simulink model "Multi_Boiler_Common_header"  (R2025b)
settings: Solver=ode15s  StartTime=0.0  StopTime=800  FixedStep=1000  RelTol=1e-2
values from neighbouring files (symbols this model uses):
  Adc = 0.7    [Init_two_Boilers.m]
  b = 0.030    (= 0.03)    [Init_two_Boilers.m]
  k1 = (2 * rho_w1 * Adc * (rho_w1 - rho_s1) * g * a7_1 * Vr) / max(q_dc^2, 1e-12)    [Init_two_Boilers.m]
  k2 = (2 * rho_w2 * Adc * (rho_w2 - rho_s2) * g * a7_2 * Vr) / max(q_dc^2, 1e-12)    [Init_two_Boilers.m]
  m_metal = 1e6    (= 1000000)    [Init_two_Boilers.m]
  m_riser = 2e5    (= 200000)    [Init_two_Boilers.m]
  tau_s = 1e-2    (= 0.01)    [Init_two_Boilers.m]
  u0_1 = [Q1_MW; q_s1; q_s1; h_f]    [Init_two_Boilers.m]
  u0_2 = [Q2_MW; q_s2; q_s2; h_f]    [Init_two_Boilers.m]
  Vr = 37    [Init_two_Boilers.m]
libraries: slpidlib x4
settings Model: SimulationMode=accelerator  PacingRate=9  Creator=Zwivh  LastModifiedBy=Zwivh
settings DebuggingCC: AlgebraicLoopMsg=none

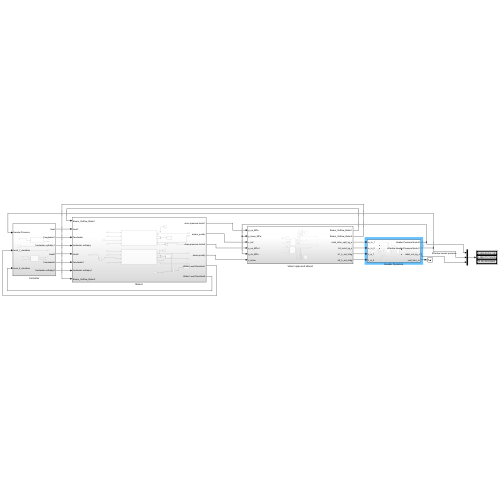
[thumbnail: Simulink's stored preview of the top-level diagram]
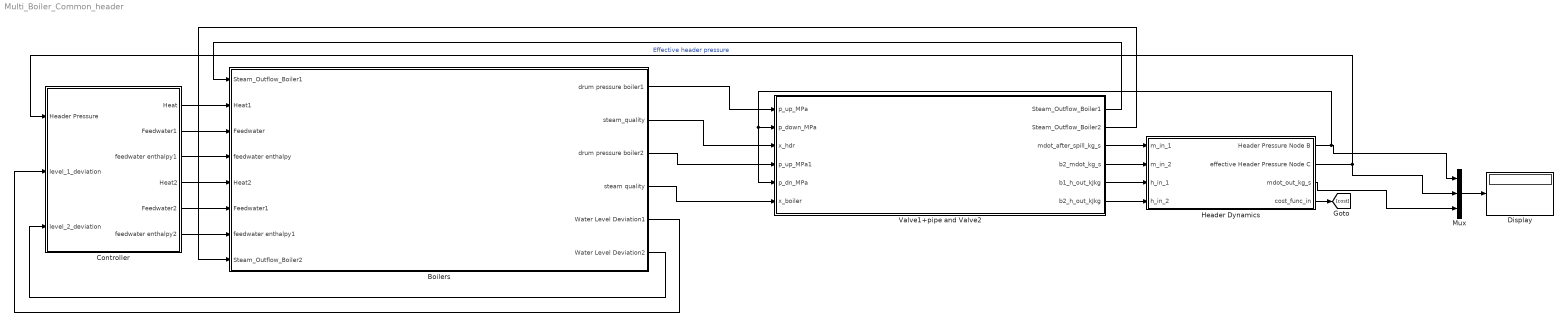
== system Multi_Boiler_Common_header ==
  Boilers : Subsystem
  Controller : Subsystem
  Display : Display
  Header Dynamics : Subsystem
  Mux : Mux  Inputs=3
  Valve1+pipe and Valve2 : Subsystem
  wires:
  Boilers/1(drum pressure boiler1) -> Valve1+pipe and Valve2/1(p_up_MPa)
  Boilers/2(steam_quality) -> Valve1+pipe and Valve2/3(x_hdr)
  Boilers/3(drum pressure boiler2) -> Valve1+pipe and Valve2/4(p_up_MPa1)
  Boilers/4(steam quality) -> Valve1+pipe and Valve2/6(x_boiler)
  Valve1+pipe and Valve2/1(Steam_Outflow_Boiler1) -> Boilers/1(Steam_Outflow_Boiler1)
  Valve1+pipe and Valve2/2(Steam_Outflow_Boiler2) -> Boilers/8(Steam_Outflow_Boiler2)
  Controller/1(Heat) -> Boilers/2(Heat1)
  Controller/2(Feedwater1) -> Boilers/3(Feedwater)
  Controller/3(feedwater enthalpy1) -> Boilers/4(feedwater enthalpy)
  Controller/4(Heat2) -> Boilers/5(Heat2)
  Controller/5(Feedwater2) -> Boilers/6(Feedwater1)
  Controller/6(feedwater enthalpy2) -> Boilers/7(feedwater enthalpy1)
  Valve1+pipe and Valve2/4(b2_mdot_kg_s) -> Header Dynamics/2(m_in_2)
  Valve1+pipe and Valve2/5(b1_h_out_kJkg) -> Header Dynamics/3(h_in_1)
  Valve1+pipe and Valve2/6(b2_h_out_kJkg) -> Header Dynamics/4(h_in_2)
  Mux/1 -> Display/1
  Header Dynamics/1(Header Pressure Node B) -> Mux/1, Valve1+pipe and Valve2/5(p_dn_MPa), Valve1+pipe and Valve2/2(p_down_MPa)
  Header Dynamics/3(mdot_out_kg_s) -> Mux/3
  Header Dynamics/2(effective Header Pressure Node C) -> Mux/2, Controller/1(Header Pressure)  "Effective header pressure"
  Header Dynamics/4(cost_func_in) -> [cost]
  Boilers/6(Water Level Deviation2) -> Controller/3(level_2_deviation)
  Boilers/5(Water Level Deviation1) -> Controller/2(level_1_deviation)
  Valve1+pipe and Valve2/3(mdot_after_spill_kg_s) -> Header Dynamics/1(m_in_1)

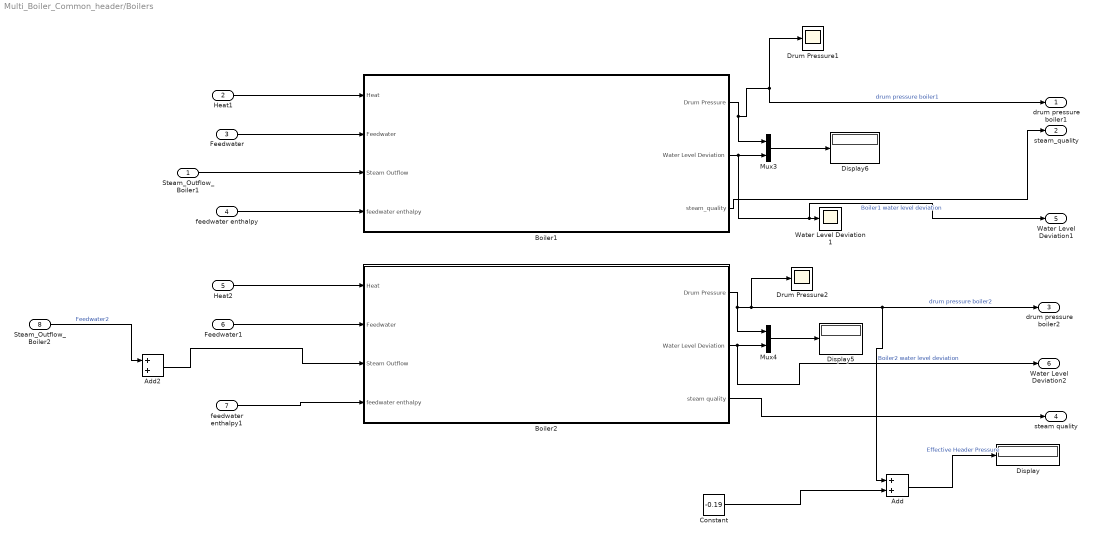
== system Multi_Boiler_Common_header/Boilers ==
  Steam_Outflow_Boiler1 : Inport
  Heat1 : Inport  Port=2
  Feedwater : Inport  Port=3
  feedwater enthalpy : Inport  Port=4
  Heat2 : Inport  Port=5
  Feedwater1 : Inport  Port=6
  feedwater enthalpy1 : Inport  Port=7
  Steam_Outflow_Boiler2 : Inport  Port=8
  Add : Sum
  Add2 : Sum
  Boiler1 : Subsystem
  Boiler2 : Subsystem
  Constant : Constant  Value=-0.19
  Display : Display
  Display5 : Display
  Display6 : Display
  Drum Pressure1 : Scope
      settings: ActiveDisplayYMinimum=2.409582484950084  ActiveDisplayYMaximum=65.31375763544925  DataLoggingVariableName=ScopeData7
  Drum Pressure2 : Scope
      settings: DataLoggingVariableName=ScopeData11
  Mux3 : Mux  Inputs=2
  Mux4 : Mux  Inputs=2
  Water Level Deviation 1 : Scope
      settings: DataLoggingVariableName=ScopeData10
  drum pressure boiler1 : Outport
  steam_quality : Outport  Port=2
  drum pressure boiler2 : Outport  Port=3
  steam quality : Outport  Port=4
  Water Level Deviation1 : Outport  Port=5
  Water Level Deviation2 : Outport  Port=6
  wires:
  Feedwater/1 -> Boiler1/2(Feedwater)
  Boiler1/1(Drum Pressure) -> Mux3/1, drum pressure boiler1/1, Drum Pressure1/1  "drum pressure boiler1"
  Boiler1/2(Water Level Deviation) -> Water Level Deviation1/1, Water Level Deviation 1/1, Mux3/2  "Boiler1 water level deviation"
  Steam_Outflow_Boiler1/1 -> Boiler1/3(Steam Outflow)
  Boiler2/2(Water Level Deviation) -> Water Level Deviation2/1, Mux4/2  "Boiler2 water level deviation"
  Mux3/1 -> Display6/1
  Feedwater1/1 -> Boiler2/2(Feedwater)
  feedwater enthalpy/1 -> Boiler1/4(feedwater enthalpy)
  Mux4/1 -> Display5/1
  Boiler2/3(steam quality) -> steam quality/1
  Boiler2/1(Drum Pressure) -> Mux4/1, Add/1, drum pressure boiler2/1, Drum Pressure2/1  "drum pressure boiler2"
  feedwater enthalpy1/1 -> Boiler2/4(feedwater enthalpy)
  Heat2/1 -> Boiler2/1(Heat)
  Heat1/1 -> Boiler1/1(Heat)
  Boiler1/3(steam_quality) -> steam_quality/1
  Add2/1 -> Boiler2/3(Steam Outflow)
  Steam_Outflow_Boiler2/1 -> Add2/1  "Feedwater2"
  Constant/1 -> Add/2
  Add/1 -> Display/1  "Effective Header Pressure"

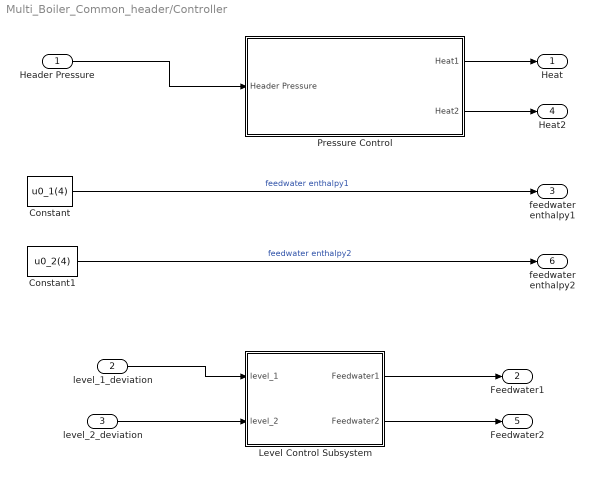
== system Multi_Boiler_Common_header/Controller ==
  Header Pressure : Inport
  level_1_deviation : Inport  Port=2
  level_2_deviation : Inport  Port=3
  Constant : Constant  Value=u0_1(4)
  Constant1 : Constant  Value=u0_2(4)
  Level Control Subsystem : Subsystem
  Pressure Control : Subsystem
  Heat : Outport
  Feedwater1 : Outport  Port=2
  feedwater enthalpy1 : Outport  Port=3
  Heat2 : Outport  Port=4
  Feedwater2 : Outport  Port=5
  feedwater enthalpy2 : Outport  Port=6
  wires:
  Constant1/1 -> feedwater enthalpy2/1  "feedwater enthalpy2"
  Constant/1 -> feedwater enthalpy1/1  "feedwater enthalpy1"
  Pressure Control/1(Heat1) -> Heat/1
  Pressure Control/2(Heat2) -> Heat2/1
  Level Control Subsystem/1(Feedwater1) -> Feedwater1/1
  Level Control Subsystem/2(Feedwater2) -> Feedwater2/1
  Header Pressure/1 -> Pressure Control/1(Header Pressure)
  level_2_deviation/1 -> Level Control Subsystem/2(level_2)
  level_1_deviation/1 -> Level Control Subsystem/1(level_1)

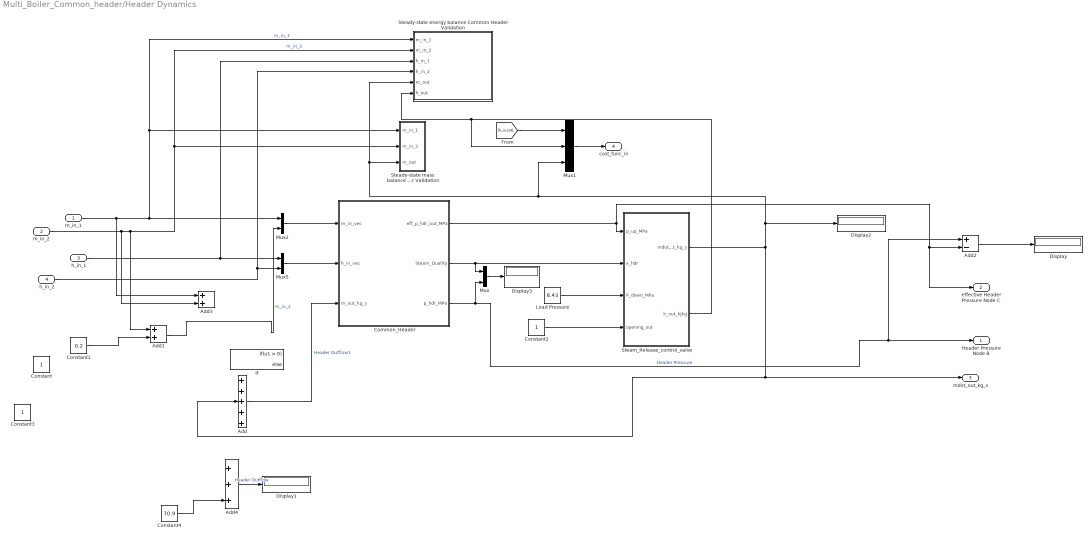
== system Multi_Boiler_Common_header/Header Dynamics ==
  m_in_1 : Inport
  m_in_2 : Inport  Port=2
  h_in_1 : Inport  Port=3
  h_in_2 : Inport  Port=4
  Add : Sum  Inputs=+++++
  Add1 : Sum
  Add2 : Sum  Inputs=+-
  Add3 : Sum
  Add4 : Sum  Inputs=+++
  Common_Header : Subsystem
  Constant : Constant
  Constant1 : Constant  Value=0.2
  Constant2 : Constant
  Constant3 : Constant
  Constant4 : Constant  Value=70.9
  Display{,1..3} (4 alike) : Display
  If : If
  Load Pressure : Constant  Value=8.43
  Mux : Mux  Inputs=2
  Mux1 : Mux  Inputs=3
  Mux2 : Mux  Inputs=2
  Mux5 : Mux  Inputs=2
  Steady‑state energy balance Common Header Validation : Subsystem
  Steady‑state mass balance Common Header Validation : Subsystem
  "Steam_Release_control_valve " : Subsystem
  Header Pressure Node B : Outport
  effective Header Pressure Node C : Outport  Port=2
  mdot_out_kg_s : Outport  Port=3
  cost_func_in : Outport  Port=4
  wires:
  Mux2/1 -> Common_Header/1(m_in_vec)
  Common_Header/2(Steam_Quality) -> Mux/1, "Steam_Release_control_valve "/2(x_hdr)
  "Steam_Release_control_valve "/2(h_out_kJkg) -> Mux1/2, Steady‑state energy balance Common Header Validation/6(h_out)
  m_in_1/1 -> Add3/1, Mux2/1, Steady‑state energy balance Common Header Validation/1(m_in_1), Steady‑state mass balance Common Header Validation/1(m_in_1)  "m_in_1"
  Mux5/1 -> Common_Header/2(h_in_vec)
  Load Pressure/1 -> "Steam_Release_control_valve "/3(P_down_MPa)
  Add/1 -> Common_Header/3(m_out_kg_s)  "Header Outflow1"
  Constant2/1 -> "Steam_Release_control_valve "/4(opening_out)
  h_in_1/1 -> Mux5/1, Steady‑state energy balance Common Header Validation/3(h_in_1)
  h_in_2/1 -> Mux5/2, Steady‑state energy balance Common Header Validation/4(h_in_2)
  m_in_2/1 -> Add3/2, Add1/1, Steady‑state energy balance Common Header Validation/2(m_in_2), Steady‑state mass balance Common Header Validation/2(m_in_2)  "m_in_2"
  Common_Header/1(eff_p_hdr_out_MPa) -> "Steam_Release_control_valve "/1(p_up_MPa), Add2/2, effective Header Pressure Node C/1
  Common_Header/3(p_hdr_MPa) -> Mux/2, Add2/1, Header Pressure Node B/1  "Header Pressure"
  Add2/1 -> Display/1
  Mux/1 -> Display3/1
  Mux1/1 -> cost_func_in/1
  [h_in_tot] -> Mux1/1
  Constant1/1 -> Add1/2
  Add1/1 -> Mux2/2  "m_in_2"
  "Steam_Release_control_valve "/1(mdot_out_kg_s) -> mdot_out_kg_s/1, Add/3, Mux1/3, Steady‑state energy balance Common Header Validation/5(m_out), Steady‑state mass balance Common Header Validation/3(m_out), Display2/1
  Constant4/1 -> Add4/3
  Add4/1 -> Display1/1  "Header Outflow"

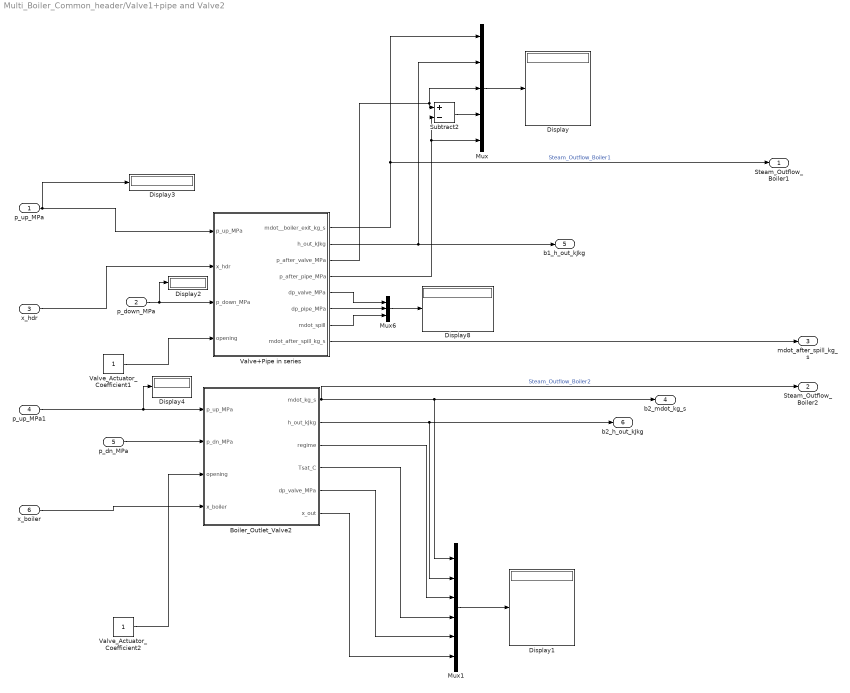
== system Multi_Boiler_Common_header/Valve1+pipe and Valve2 ==
  p_up_MPa : Inport
  p_down_MPa : Inport  Port=2
  x_hdr : Inport  Port=3
  p_up_MPa1 : Inport  Port=4
  p_dn_MPa : Inport  Port=5
  x_boiler : Inport  Port=6
  Boiler_Outlet_Valve2 : Subsystem
  Display{,1..4,8} (6 alike) : Display
  Mux : Mux  Inputs=5
  Mux1 : Mux  Inputs=6
  Mux6 : Mux  Inputs=3
  Subtract2 : Sum  Inputs=+-
  Valve+Pipe in series : Subsystem
  Valve_Actuator_Coefficient1 : Constant
  Valve_Actuator_Coefficient2 : Constant
  Steam_Outflow_Boiler1 : Outport
  Steam_Outflow_Boiler2 : Outport  Port=2
  mdot_after_spill_kg_s : Outport  Port=3
  b2_mdot_kg_s : Outport  Port=4
  b1_h_out_kJkg : Outport  Port=5
  b2_h_out_kJkg : Outport  Port=6
  wires:
  x_hdr/1 -> Valve+Pipe in series/2(x_hdr)
  Boiler_Outlet_Valve2/4(Tsat_C) -> Mux1/4
  Valve+Pipe in series/1(mdot__boiler_exit_kg_s) -> Mux/1, Steam_Outflow_Boiler1/1  "Steam_Outflow_Boiler1"
  Valve+Pipe in series/5(dp_valve_MPa) -> Mux6/1
  x_boiler/1 -> Boiler_Outlet_Valve2/4(x_boiler)
  Valve+Pipe in series/3(p_after_valve_MPa) -> Mux/3, Subtract2/1
  Valve+Pipe in series/4(p_after_pipe_MPa) -> Subtract2/2, Mux/5
  Valve_Actuator_Coefficient2/1 -> Boiler_Outlet_Valve2/3(opening)
  Mux1/1 -> Display1/1
  Boiler_Outlet_Valve2/2(h_out_kJkg) -> b2_h_out_kJkg/1, Mux1/2
  Mux/1 -> Display/1
  Boiler_Outlet_Valve2/6(x_out) -> Mux1/6
  Valve_Actuator_Coefficient1/1 -> Valve+Pipe in series/4(opening)
  Boiler_Outlet_Valve2/3(regime) -> Mux1/3
  Boiler_Outlet_Valve2/1(mdot_kg_s) -> b2_mdot_kg_s/1, Mux1/1, Steam_Outflow_Boiler2/1  "Steam_Outflow_Boiler2"
  Mux6/1 -> Display8/1
  Boiler_Outlet_Valve2/5(dp_valve_MPa) -> Mux1/5
  Subtract2/1 -> Mux/4
  Valve+Pipe in series/6(dp_pipe_MPa) -> Mux6/2
  Valve+Pipe in series/7(mdot_spill) -> Mux6/3
  Valve+Pipe in series/2(h_out_kJkg) -> b1_h_out_kJkg/1, Mux/2
  p_dn_MPa/1 -> Boiler_Outlet_Valve2/2(p_dn_MPa)
  p_down_MPa/1 -> Display2/1, Valve+Pipe in series/3(p_down_MPa)
  p_up_MPa/1 -> Display3/1, Valve+Pipe in series/1(p_up_MPa)
  p_up_MPa1/1 -> Display4/1, Boiler_Outlet_Valve2/1(p_up_MPa)
  Valve+Pipe in series/8(mdot_after_spill_kg_s) -> mdot_after_spill_kg_s/1

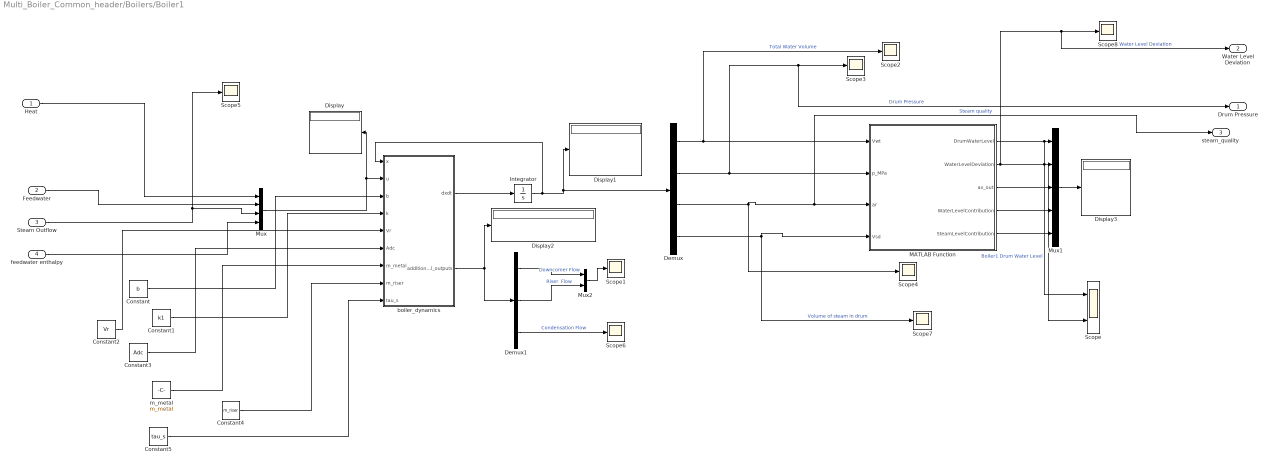
== system Multi_Boiler_Common_header/Boilers/Boiler1 ==
  Heat : Inport
  Feedwater : Inport  Port=2
  Steam Outflow : Inport  Port=3
  feedwater enthalpy : Inport  Port=4
  Constant : Constant  Value=b
  Constant1 : Constant  Value=k1
  Constant2 : Constant  Value=Vr
  Constant3 : Constant  Value=Adc
  Constant4 : Constant  Value=m_riser
  Constant5 : Constant  Value=tau_s
  Demux : Demux
  Demux1 : Demux  Outputs=3
  Display{,1..3} (4 alike) : Display
  Integrator : Integrator  InitialCondition=[57.8;8.8;0.083;4.9]
  MATLAB Function : MATLAB Function  TreatAsAtomicUnit=on
  Mux : Mux
  Mux1 : Mux  Inputs=5
  Mux2 : Mux  Inputs=2
  Scope : Scope  NumInputPorts=2
      settings: ActiveDisplayYMinimum=-0.11553187271684388  ActiveDisplayYMaximum=0.97989716685186512  DataLoggingVariableName=ScopeData9
  Scope{1..8} (8 alike) : Scope
      Scope1 settings: ActiveDisplayYMinimum=1149.8937170235527  ActiveDisplayYMaximum=1360.0825647224879  DataLoggingVariableName=ScopeData6
      Scope3 settings: ActiveDisplayYMinimum=5.1731172032500083  ActiveDisplayYMaximum=8.869653644083332
      Scope4 settings: DataLoggingVariableName=ScopeData2
      Scope5 settings: ActiveDisplayYMinimum=81.783639946245515  ActiveDisplayYMaximum=87.68969538020076  DataLoggingVariableName=ScopeData3
      Scope6 settings: DataLoggingVariableName=ScopeData4
      Scope7 settings: DataLoggingVariableName=ScopeData5
      Scope8 settings: ActiveDisplayYMinimum=-0.31931831052985321  ActiveDisplayYMaximum=0.12332586369569878  DataLoggingVariableName=ScopeData8
  boiler_dynamics : MATLAB Function  TreatAsAtomicUnit=on
  "m_metal " : Constant  Value=m_metal
  Drum Pressure : Outport
  Water Level Deviation : Outport  Port=2
  steam_quality : Outport  Port=3
  wires:
  MATLAB Function/3(av_out) -> Mux1/3
  Steam Outflow/1 -> Scope5/1, Mux/3
  Integrator/1 -> Display1/1, Demux/1, boiler_dynamics/1(x)
  Constant4/1 -> boiler_dynamics/8(m_riser)
  Demux/1 -> Scope2/1, MATLAB Function/1(Vwt)  "Total Water Volume"
  MATLAB Function/2(WaterLevelDeviation) -> Water Level Deviation/1, Scope8/1, Scope/2, Mux1/2  "Water Level Deviation"
  Demux/2 -> Drum Pressure/1, Scope3/1, MATLAB Function/2(p_MPa)  "Drum Pressure"
  Demux1/2 -> Mux2/2  "Riser  Flow"
  boiler_dynamics/2(additional_outputs) -> Display2/1, Demux1/1
  Constant2/1 -> boiler_dynamics/5(Vr)
  Demux/3 -> Scope4/1, steam_quality/1, MATLAB Function/3(ar)  "Steam quality"
  Constant3/1 -> boiler_dynamics/6(Adc)
  Mux2/1 -> Scope1/1
  Demux1/1 -> Mux2/1  "Downcomer Flow"
  Constant1/1 -> boiler_dynamics/4(k)
  Mux/1 -> Display/1, boiler_dynamics/2(u)
  MATLAB Function/5(SteamLevelContribution) -> Mux1/5
  MATLAB Function/1(DrumWaterLevel) -> Scope/1, Mux1/1  "Boiler1 Drum Water Level"
  Constant/1 -> boiler_dynamics/3(b)
  "m_metal "/1 -> boiler_dynamics/7(m_metal)
  Demux/4 -> Scope7/1, MATLAB Function/4(Vsd)  "Volume of steam in drum"
  Constant5/1 -> boiler_dynamics/9(tau_s)
  Heat/1 -> Mux/1
  boiler_dynamics/1(dxdt) -> Integrator/1
  Demux1/3 -> Scope6/1  "Condensation Flow"
  MATLAB Function/4(WaterLevelContribution) -> Mux1/4
  Mux1/1 -> Display3/1
  Feedwater/1 -> Mux/2
  feedwater enthalpy/1 -> Mux/4

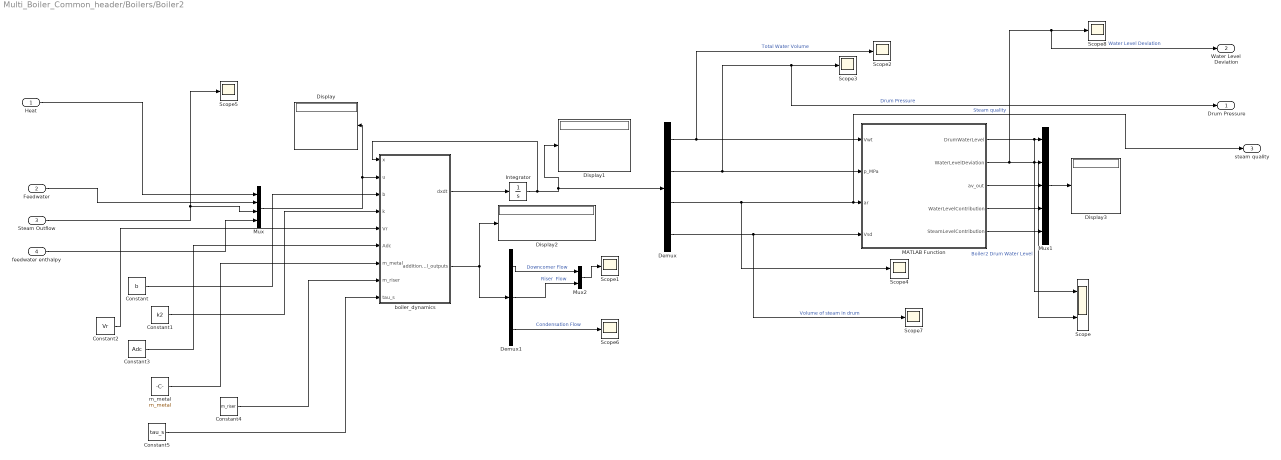
== system Multi_Boiler_Common_header/Boilers/Boiler2 ==
  Heat : Inport
  Feedwater : Inport  Port=2
  Steam Outflow : Inport  Port=3
  feedwater enthalpy : Inport  Port=4
  Constant : Constant  Value=b
  Constant1 : Constant  Value=k2
  Constant2 : Constant  Value=Vr
  Constant3 : Constant  Value=Adc
  Constant4 : Constant  Value=m_riser
  Constant5 : Constant  Value=tau_s
  Demux : Demux
  Demux1 : Demux  Outputs=3
  Display{,1..3} (4 alike) : Display
  Integrator : Integrator  InitialCondition=[57.6;8.69;0.066;4.9]
  MATLAB Function : MATLAB Function  TreatAsAtomicUnit=on
  Mux : Mux
  Mux1 : Mux  Inputs=5
  Mux2 : Mux  Inputs=2
  Scope : Scope  NumInputPorts=2
      settings: ActiveDisplayYMinimum=-0.43318786127461034  ActiveDisplayYMaximum=1.0681425276889893  DataLoggingVariableName=ScopeData9
  Scope{1..8} (8 alike) : Scope
      Scope1 settings: ActiveDisplayYMinimum=1149.8937170235527  ActiveDisplayYMaximum=1360.0825647224879  DataLoggingVariableName=ScopeData6
      Scope3 settings: ActiveDisplayYMinimum=7.2515160346094891  ActiveDisplayYMaximum=9.62463808005422
      Scope4 settings: DataLoggingVariableName=ScopeData2
      Scope5 settings: ActiveDisplayYMinimum=81.783639946245515  ActiveDisplayYMaximum=87.68969538020076  DataLoggingVariableName=ScopeData3
      Scope6 settings: DataLoggingVariableName=ScopeData4
      Scope7 settings: DataLoggingVariableName=ScopeData5
      Scope8 settings: ActiveDisplayYMinimum=-0.1700298535717597  ActiveDisplayYMaximum=0.091752188934218326  DataLoggingVariableName=ScopeData8
  boiler_dynamics : MATLAB Function  TreatAsAtomicUnit=on
  "m_metal " : Constant  Value=m_metal
  Drum Pressure : Outport
  Water Level Deviation : Outport  Port=2
  steam quality : Outport  Port=3
  wires:
  MATLAB Function/3(av_out) -> Mux1/3
  Steam Outflow/1 -> Scope5/1, Mux/3
  Integrator/1 -> Display1/1, Demux/1, boiler_dynamics/1(x)
  Constant4/1 -> boiler_dynamics/8(m_riser)
  Demux/1 -> Scope2/1, MATLAB Function/1(Vwt)  "Total Water Volume"
  MATLAB Function/2(WaterLevelDeviation) -> Water Level Deviation/1, Scope8/1, Scope/2, Mux1/2  "Water Level Deviation"
  Demux/2 -> Drum Pressure/1, Scope3/1, MATLAB Function/2(p_MPa)  "Drum Pressure"
  Demux1/2 -> Mux2/2  "Riser  Flow"
  boiler_dynamics/2(additional_outputs) -> Display2/1, Demux1/1
  Constant2/1 -> boiler_dynamics/5(Vr)
  Demux/3 -> Scope4/1, steam quality/1, MATLAB Function/3(ar)  "Steam quality"
  Constant3/1 -> boiler_dynamics/6(Adc)
  Mux2/1 -> Scope1/1
  Demux1/1 -> Mux2/1  "Downcomer Flow"
  Constant1/1 -> boiler_dynamics/4(k)
  Mux/1 -> Display/1, boiler_dynamics/2(u)
  MATLAB Function/5(SteamLevelContribution) -> Mux1/5
  MATLAB Function/1(DrumWaterLevel) -> Scope/1, Mux1/1  "Boiler2 Drum Water Level"
  Constant/1 -> boiler_dynamics/3(b)
  "m_metal "/1 -> boiler_dynamics/7(m_metal)
  Demux/4 -> Scope7/1, MATLAB Function/4(Vsd)  "Volume of steam in drum"
  Constant5/1 -> boiler_dynamics/9(tau_s)
  Heat/1 -> Mux/1
  boiler_dynamics/1(dxdt) -> Integrator/1
  Demux1/3 -> Scope6/1  "Condensation Flow"
  MATLAB Function/4(WaterLevelContribution) -> Mux1/4
  Mux1/1 -> Display3/1
  Feedwater/1 -> Mux/2
  feedwater enthalpy/1 -> Mux/4

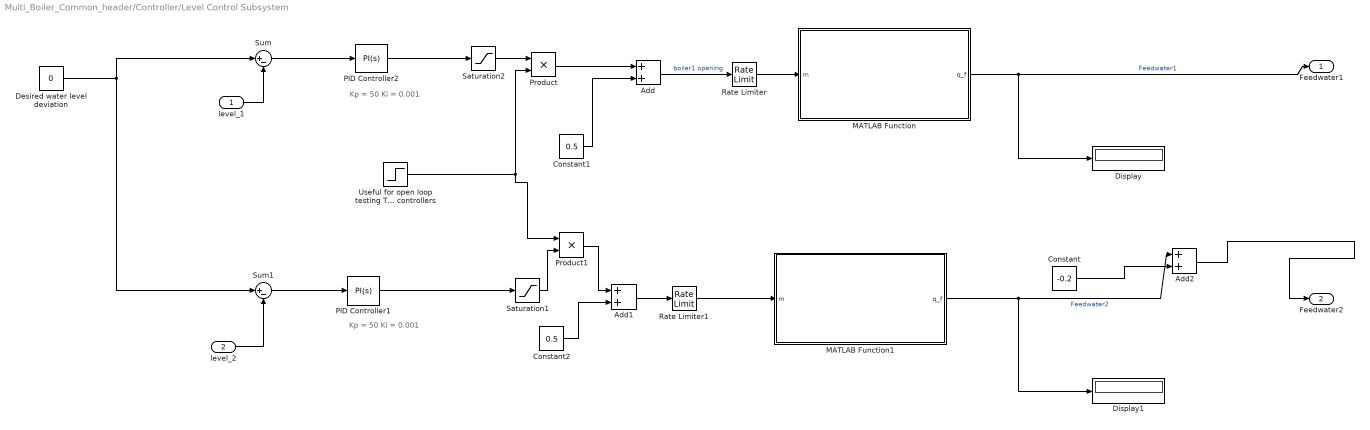
== system Multi_Boiler_Common_header/Controller/Level Control Subsystem ==
  note: Kp = 50
      | Ki = 0.001
  note: Kp = 50
      | Ki = 0.001
  level_1 : Inport
  level_2 : Inport  Port=2
  Add : Sum
  Add1 : Sum
  Add2 : Sum
  Constant : Constant  Value=-0.2
  Constant1 : Constant  Value=0.5
  Constant2 : Constant  Value=0.5
  "Desired water level deviation " : Constant  Value=0
  Display : Display
  Display1 : Display
  MATLAB Function : MATLAB Function  TreatAsAtomicUnit=on
  MATLAB Function1 : MATLAB Function  TreatAsAtomicUnit=on
  PID Controller1 : slpidlib/PID Controller  Controller=PI  Form=Parallel  TimeDomain=Continuous-time  UseExternalTs=off  SampleTime=5  IntegratorMethod=Forward Euler  FilterMethod=Forward Euler  ControllerParametersSource=internal  P=0.5e2  I=1e-3  UseKiTs=off  D=1  UseExternalDerivativeSource=off  N=100  UseFilter=on  TunerSelectOption=Transfer Function Based (PID Tuner App)  InitialConditionSource=internal  InitialConditionForIntegrator=0  InitialConditionForFilter=0  DifferentiatorICPrevScaledInput=0  ExternalReset=none  TrackingMode=off  Kt=1  LimitOutput=off  SatLimitsSource=internal  UpperSaturationLimit=inf  LowerSaturationLimit=-inf  LinearizeAsGain=on  AntiWindupMode=none  Kb=1  LimitIntegrator=off  UpperIntegratorSaturationLimit=inf  LowerIntegratorSaturationLimit=-inf  POutMin=[]  POutMax=[]  IOutMin=[]  IOutMax=[]  DOutMin=[]  DOutMax=[]  NOutMin=[]  NOutMax=[]  SumOutMin=[]  SumOutMax=[]  SaturationOutMin=[]  SaturationOutMax=[]  PParamMin=[]  PParamMax=[]  IParamMin=[]  IParamMax=[]  DParamMin=[]  DParamMax=[]  NParamMin=[]  NParamMax=[]  KbParamMin=[]  KbParamMax=[]  KtParamMin=[]  KtParamMax=[]  KbOutMin=[]  KbOutMax=[]  KtOutMin=[]  KtOutMax=[]  IntegratorOutMin=[]  IntegratorOutMax=[]  FilterOutMin=[]  FilterOutMax=[]  SumI1OutMin=[]  SumI1OutMax=[]  SumI2OutMin=[]  SumI2OutMax=[]  SumI3OutMin=[]  SumI3OutMax=[]  SumI4OutMin=[]  SumI4OutMax=[]  SumDOutMin=[]  SumDOutMax=[]  DifferentiatorOutMin=[]  DifferentiatorOutMax=[]  FilterDiffOutCoefMin=[]  FilterDiffOutCoefMax=[]  ReciprocalOutMin=[]  ReciprocalOutMax=[]  SumDenOutMin=[]  SumDenOutMax=[]  SumNumOutMin=[]  SumNumOutMax=[]  DivideOutMin=[]  DivideOutMax=[]  UdiffTsProdOutMin=[]  UdiffTsProdOutMax=[]  NTsProdOutMin=[]  NTsProdOutMax=[]  UintegralTsProdOutMin=[]  UintegralTsProdOutMax=[]  UngainTsProdOutMin=[]  UngainTsProdOutMax=[]  ClampingZeroOutDataTypeStr=Inherit: Inherit via back propagation  ClampingZeroOutMin=[]  ClampingZeroOutMax=[]  FilterDenConstantOutDataTypeStr=Inherit: Inherit via back propagation  FilterDenConstantOutMin=[]  FilterDenConstantOutMax=[]  PCopyOutDataTypeStr=Inherit: Inherit via back propagation  PCopyOutMin=[]  PCopyOutMax=[]  NCopyOutDataTypeStr=Inherit: Inherit via back propagation  NCopyOutMin=[]  NCopyOutMax=[]  IntegratorContinuousStateAttributes=''  IntegratorStateMustResolveToSignalObject=off  IntegratorRTWStateStorageClass=Auto  FilterContinuousStateAttributes=''  FilterStateMustResolveToSignalObject=off  FilterRTWStateStorageClass=Auto  ParallelPVariant=InternalParameters  IdealPVariant=Disabled  IVariant=InternalParameters  DVariant=Disabled  IntegratorVariant=Continuous  SatVariant=Disabled  AWVariant=Passthrough  PCopyVariant=Disabled  TRVariant=Disabled  FdbkBlocksVariant=Forward  IdealPFdbkVariant=Disabled  SatFdbkVariant=Disabled  DerivativeFilterVariant=Disabled  NVariant=Disabled  NCopyVariant=Disabled_SignalSpec  FilterICVariant=Disabled  IntegratorICVariant=InternalICs  ExternalResetVariant=Disabled  TRSumVariant=Passthrough  SumFdbkVariant=Disabled  SumVariant=Sum_PI  TsampFilterVariant=InternalTs  TsampNgainVariant=Passthrough  TsampIntegralVariant=Disabled_SignalSpec  ExternalSaturationOutDataTypeStr=Inherit: Same as second input  DerivativeSourceVariant=Disabled  PreIntVariant=InternalPreInt
  PID Controller2 : slpidlib/PID Controller  Controller=PI  Form=Parallel  TimeDomain=Continuous-time  UseExternalTs=off  SampleTime=5  IntegratorMethod=Forward Euler  FilterMethod=Forward Euler  ControllerParametersSource=internal  P=0.5e2  I=1e-3  UseKiTs=off  D=1  UseExternalDerivativeSource=off  N=100  UseFilter=on  TunerSelectOption=Transfer Function Based (PID Tuner App)  InitialConditionSource=internal  InitialConditionForIntegrator=0  InitialConditionForFilter=0  DifferentiatorICPrevScaledInput=0  ExternalReset=none  TrackingMode=off  Kt=1  LimitOutput=off  SatLimitsSource=internal  UpperSaturationLimit=inf  LowerSaturationLimit=-inf  LinearizeAsGain=on  AntiWindupMode=none  Kb=1  LimitIntegrator=off  UpperIntegratorSaturationLimit=inf  LowerIntegratorSaturationLimit=-inf  POutMin=[]  POutMax=[]  IOutMin=[]  IOutMax=[]  DOutMin=[]  DOutMax=[]  NOutMin=[]  NOutMax=[]  SumOutMin=[]  SumOutMax=[]  SaturationOutMin=[]  SaturationOutMax=[]  PParamMin=[]  PParamMax=[]  IParamMin=[]  IParamMax=[]  DParamMin=[]  DParamMax=[]  NParamMin=[]  NParamMax=[]  KbParamMin=[]  KbParamMax=[]  KtParamMin=[]  KtParamMax=[]  KbOutMin=[]  KbOutMax=[]  KtOutMin=[]  KtOutMax=[]  IntegratorOutMin=[]  IntegratorOutMax=[]  FilterOutMin=[]  FilterOutMax=[]  SumI1OutMin=[]  SumI1OutMax=[]  SumI2OutMin=[]  SumI2OutMax=[]  SumI3OutMin=[]  SumI3OutMax=[]  SumI4OutMin=[]  SumI4OutMax=[]  SumDOutMin=[]  SumDOutMax=[]  DifferentiatorOutMin=[]  DifferentiatorOutMax=[]  FilterDiffOutCoefMin=[]  FilterDiffOutCoefMax=[]  ReciprocalOutMin=[]  ReciprocalOutMax=[]  SumDenOutMin=[]  SumDenOutMax=[]  SumNumOutMin=[]  SumNumOutMax=[]  DivideOutMin=[]  DivideOutMax=[]  UdiffTsProdOutMin=[]  UdiffTsProdOutMax=[]  NTsProdOutMin=[]  NTsProdOutMax=[]  UintegralTsProdOutMin=[]  UintegralTsProdOutMax=[]  UngainTsProdOutMin=[]  UngainTsProdOutMax=[]  ClampingZeroOutDataTypeStr=Inherit: Inherit via back propagation  ClampingZeroOutMin=[]  ClampingZeroOutMax=[]  FilterDenConstantOutDataTypeStr=Inherit: Inherit via back propagation  FilterDenConstantOutMin=[]  FilterDenConstantOutMax=[]  PCopyOutDataTypeStr=Inherit: Inherit via back propagation  PCopyOutMin=[]  PCopyOutMax=[]  NCopyOutDataTypeStr=Inherit: Inherit via back propagation  NCopyOutMin=[]  NCopyOutMax=[]  IntegratorContinuousStateAttributes=''  IntegratorStateMustResolveToSignalObject=off  IntegratorRTWStateStorageClass=Auto  FilterContinuousStateAttributes=''  FilterStateMustResolveToSignalObject=off  FilterRTWStateStorageClass=Auto  ParallelPVariant=InternalParameters  IdealPVariant=Disabled  IVariant=InternalParameters  DVariant=Disabled  IntegratorVariant=Continuous  SatVariant=Disabled  AWVariant=Passthrough  PCopyVariant=Disabled  TRVariant=Disabled  FdbkBlocksVariant=Forward  IdealPFdbkVariant=Disabled  SatFdbkVariant=Disabled  DerivativeFilterVariant=Disabled  NVariant=Disabled  NCopyVariant=Disabled_SignalSpec  FilterICVariant=Disabled  IntegratorICVariant=InternalICs  ExternalResetVariant=Disabled  TRSumVariant=Passthrough  SumFdbkVariant=Disabled  SumVariant=Sum_PI  TsampFilterVariant=InternalTs  TsampNgainVariant=Passthrough  TsampIntegralVariant=Disabled_SignalSpec  ExternalSaturationOutDataTypeStr=Inherit: Same as second input  DerivativeSourceVariant=Disabled  PreIntVariant=InternalPreInt
  Product : Product
  Product1 : Product
  Rate Limiter : RateLimiter  RisingSlewLimit=0.03  FallingSlewLimit=-0.03  SampleTimeMode=inherited
  Rate Limiter1 : RateLimiter  RisingSlewLimit=0.03  FallingSlewLimit=-0.03  SampleTimeMode=inherited
  Saturation1 : Saturate
  Saturation2 : Saturate
  Sum : Sum  Inputs=|+-
  Sum1 : Sum  Inputs=|+-
  Useful for open loop testing Turn On/Off the controllers : Step  Time=0  After=0  SampleTime=0
  Feedwater1 : Outport
  Feedwater2 : Outport  Port=2
  wires:
  Rate Limiter1/1 -> MATLAB Function1/1(m)
  MATLAB Function1/1(q_f) -> Add2/1, Display1/1  "Feedwater2"
  Add/1 -> Rate Limiter/1  "boiler1 opening"
  Add1/1 -> Rate Limiter1/1
  Rate Limiter/1 -> MATLAB Function/1(m)
  Constant1/1 -> Add/2
  MATLAB Function/1(q_f) -> Feedwater1/1, Display/1  "Feedwater1"
  Saturation1/1 -> Product1/2
  Constant2/1 -> Add1/2
  Sum/1 -> PID Controller2/1
  Sum1/1 -> PID Controller1/1
  level_2/1 -> Sum1/2
  Useful for open loop testing Turn On/Off the controllers/1 -> Product1/1, Product/2
  Saturation2/1 -> Product/1
  Product/1 -> Add/1
  level_1/1 -> Sum/2
  PID Controller1/1 -> Saturation1/1
  PID Controller2/1 -> Saturation2/1
  "Desired water level deviation "/1 -> Sum/1, Sum1/1
  Product1/1 -> Add1/1
  Constant/1 -> Add2/2
  Add2/1 -> Feedwater2/1

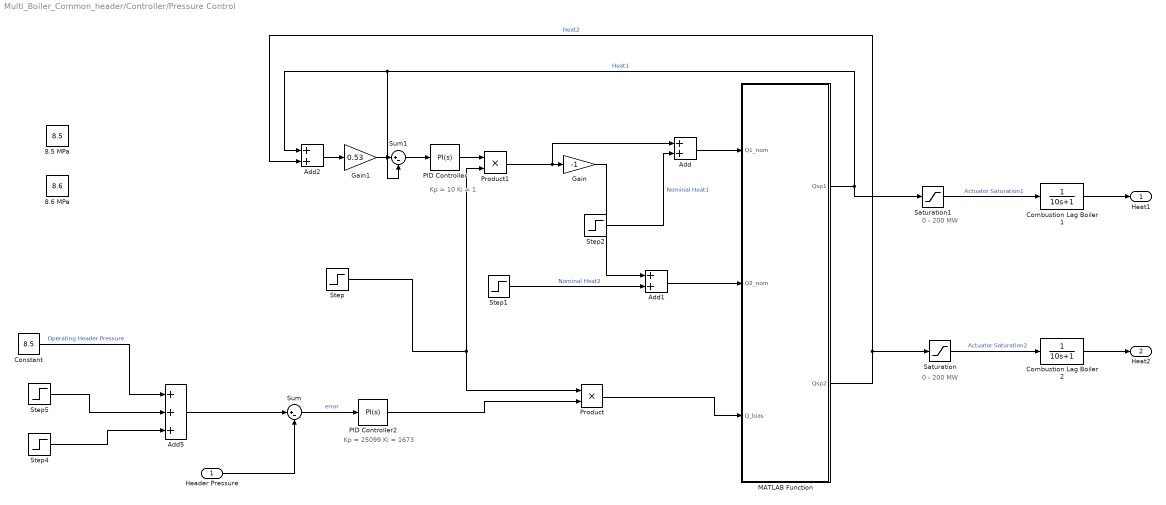
== system Multi_Boiler_Common_header/Controller/Pressure Control ==
  note: Kp = 25099
      | Ki = 1673
  note: Kp = 10
      | Ki = 1
  note: 0 - 200 MW
  note: 0 - 200 MW
  Header Pressure : Inport
  8.5 MPa : Constant  Value=8.5
  8.6 MPa : Constant  Value=8.6
  Add : Sum
  Add1 : Sum
  Add2 : Sum
  Add5 : Sum  Inputs=+++
  Combustion Lag Boiler 1 : TransferFcn  Denominator=[10 1]
  Combustion Lag Boiler 2 : TransferFcn  Denominator=[10 1]
  Constant : Constant  Value=8.5
  Gain : Gain  Gain=-1
  Gain1 : Gain  Gain=0.53
  MATLAB Function : MATLAB Function  TreatAsAtomicUnit=on
  PID Controller : slpidlib/PID Controller  Controller=PI  Form=Parallel  TimeDomain=Continuous-time  UseExternalTs=off  SampleTime=10  IntegratorMethod=Forward Euler  FilterMethod=Forward Euler  ControllerParametersSource=internal  P=10  I=0.076  UseKiTs=off  D=0  UseExternalDerivativeSource=off  N=100  UseFilter=on  TunerSelectOption=Transfer Function Based (PID Tuner App)  InitialConditionSource=internal  InitialConditionForIntegrator=0  InitialConditionForFilter=0  DifferentiatorICPrevScaledInput=0  ExternalReset=none  TrackingMode=off  Kt=1  LimitOutput=off  SatLimitsSource=internal  UpperSaturationLimit=inf  LowerSaturationLimit=-inf  LinearizeAsGain=on  AntiWindupMode=none  Kb=1  LimitIntegrator=off  UpperIntegratorSaturationLimit=inf  LowerIntegratorSaturationLimit=-inf  POutMin=[]  POutMax=[]  IOutMin=[]  IOutMax=[]  DOutMin=[]  DOutMax=[]  NOutMin=[]  NOutMax=[]  SumOutMin=[]  SumOutMax=[]  SaturationOutMin=[]  SaturationOutMax=[]  PParamMin=[]  PParamMax=[]  IParamMin=[]  IParamMax=[]  DParamMin=[]  DParamMax=[]  NParamMin=[]  NParamMax=[]  KbParamMin=[]  KbParamMax=[]  KtParamMin=[]  KtParamMax=[]  KbOutMin=[]  KbOutMax=[]  KtOutMin=[]  KtOutMax=[]  IntegratorOutMin=[]  IntegratorOutMax=[]  FilterOutMin=[]  FilterOutMax=[]  SumI1OutMin=[]  SumI1OutMax=[]  SumI2OutMin=[]  SumI2OutMax=[]  SumI3OutMin=[]  SumI3OutMax=[]  SumI4OutMin=[]  SumI4OutMax=[]  SumDOutMin=[]  SumDOutMax=[]  DifferentiatorOutMin=[]  DifferentiatorOutMax=[]  FilterDiffOutCoefMin=[]  FilterDiffOutCoefMax=[]  ReciprocalOutMin=[]  ReciprocalOutMax=[]  SumDenOutMin=[]  SumDenOutMax=[]  SumNumOutMin=[]  SumNumOutMax=[]  DivideOutMin=[]  DivideOutMax=[]  UdiffTsProdOutMin=[]  UdiffTsProdOutMax=[]  NTsProdOutMin=[]  NTsProdOutMax=[]  UintegralTsProdOutMin=[]  UintegralTsProdOutMax=[]  UngainTsProdOutMin=[]  UngainTsProdOutMax=[]  ClampingZeroOutDataTypeStr=Inherit: Inherit via back propagation  ClampingZeroOutMin=[]  ClampingZeroOutMax=[]  FilterDenConstantOutDataTypeStr=Inherit: Inherit via back propagation  FilterDenConstantOutMin=[]  FilterDenConstantOutMax=[]  PCopyOutDataTypeStr=Inherit: Inherit via back propagation  PCopyOutMin=[]  PCopyOutMax=[]  NCopyOutDataTypeStr=Inherit: Inherit via back propagation  NCopyOutMin=[]  NCopyOutMax=[]  IntegratorContinuousStateAttributes=''  IntegratorStateMustResolveToSignalObject=off  IntegratorRTWStateStorageClass=Auto  FilterContinuousStateAttributes=''  FilterStateMustResolveToSignalObject=off  FilterRTWStateStorageClass=Auto  ParallelPVariant=InternalParameters  IdealPVariant=Disabled  IVariant=InternalParameters  DVariant=Disabled  IntegratorVariant=Continuous  SatVariant=Disabled  AWVariant=Passthrough  PCopyVariant=Disabled  TRVariant=Disabled  FdbkBlocksVariant=Forward  IdealPFdbkVariant=Disabled  SatFdbkVariant=Disabled  DerivativeFilterVariant=Disabled  NVariant=Disabled  NCopyVariant=Disabled_SignalSpec  FilterICVariant=Disabled  IntegratorICVariant=InternalICs  ExternalResetVariant=Disabled  TRSumVariant=Passthrough  SumFdbkVariant=Disabled  SumVariant=Sum_PI  TsampFilterVariant=InternalTs  TsampNgainVariant=Passthrough  TsampIntegralVariant=Disabled_SignalSpec  ExternalSaturationOutDataTypeStr=Inherit: Same as second input  DerivativeSourceVariant=Disabled  PreIntVariant=InternalPreInt
  PID Controller2 : slpidlib/PID Controller  Controller=PI  Form=Parallel  TimeDomain=Continuous-time  UseExternalTs=off  SampleTime=-1  IntegratorMethod=Forward Euler  FilterMethod=Forward Euler  ControllerParametersSource=internal  P=20763  I=1384  UseKiTs=off  D=69210  UseExternalDerivativeSource=off  N=100  UseFilter=on  TunerSelectOption=Transfer Function Based (PID Tuner App)  InitialConditionSource=internal  InitialConditionForIntegrator=0  InitialConditionForFilter=0  DifferentiatorICPrevScaledInput=0  ExternalReset=none  TrackingMode=off  Kt=1  LimitOutput=off  SatLimitsSource=internal  UpperSaturationLimit=inf  LowerSaturationLimit=-inf  LinearizeAsGain=on  AntiWindupMode=none  Kb=1  LimitIntegrator=off  UpperIntegratorSaturationLimit=inf  LowerIntegratorSaturationLimit=-inf  POutMin=[]  POutMax=[]  IOutMin=[]  IOutMax=[]  DOutMin=[]  DOutMax=[]  NOutMin=[]  NOutMax=[]  SumOutMin=[]  SumOutMax=[]  SaturationOutMin=[]  SaturationOutMax=[]  PParamMin=[]  PParamMax=[]  IParamMin=[]  IParamMax=[]  DParamMin=[]  DParamMax=[]  NParamMin=[]  NParamMax=[]  KbParamMin=[]  KbParamMax=[]  KtParamMin=[]  KtParamMax=[]  KbOutMin=[]  KbOutMax=[]  KtOutMin=[]  KtOutMax=[]  IntegratorOutMin=[]  IntegratorOutMax=[]  FilterOutMin=[]  FilterOutMax=[]  SumI1OutMin=[]  SumI1OutMax=[]  SumI2OutMin=[]  SumI2OutMax=[]  SumI3OutMin=[]  SumI3OutMax=[]  SumI4OutMin=[]  SumI4OutMax=[]  SumDOutMin=[]  SumDOutMax=[]  DifferentiatorOutMin=[]  DifferentiatorOutMax=[]  FilterDiffOutCoefMin=[]  FilterDiffOutCoefMax=[]  ReciprocalOutMin=[]  ReciprocalOutMax=[]  SumDenOutMin=[]  SumDenOutMax=[]  SumNumOutMin=[]  SumNumOutMax=[]  DivideOutMin=[]  DivideOutMax=[]  UdiffTsProdOutMin=[]  UdiffTsProdOutMax=[]  NTsProdOutMin=[]  NTsProdOutMax=[]  UintegralTsProdOutMin=[]  UintegralTsProdOutMax=[]  UngainTsProdOutMin=[]  UngainTsProdOutMax=[]  ClampingZeroOutDataTypeStr=Inherit: Inherit via back propagation  ClampingZeroOutMin=[]  ClampingZeroOutMax=[]  FilterDenConstantOutDataTypeStr=Inherit: Inherit via back propagation  FilterDenConstantOutMin=[]  FilterDenConstantOutMax=[]  PCopyOutDataTypeStr=Inherit: Inherit via back propagation  PCopyOutMin=[]  PCopyOutMax=[]  NCopyOutDataTypeStr=Inherit: Inherit via back propagation  NCopyOutMin=[]  NCopyOutMax=[]  IntegratorContinuousStateAttributes=''  IntegratorStateMustResolveToSignalObject=off  IntegratorRTWStateStorageClass=Auto  FilterContinuousStateAttributes=''  FilterStateMustResolveToSignalObject=off  FilterRTWStateStorageClass=Auto  ParallelPVariant=InternalParameters  IdealPVariant=Disabled  IVariant=InternalParameters  DVariant=Disabled  IntegratorVariant=Continuous  SatVariant=Disabled  AWVariant=Passthrough  PCopyVariant=Disabled  TRVariant=Disabled  FdbkBlocksVariant=Forward  IdealPFdbkVariant=Disabled  SatFdbkVariant=Disabled  DerivativeFilterVariant=Disabled  NVariant=Disabled  NCopyVariant=Disabled_SignalSpec  FilterICVariant=Disabled  IntegratorICVariant=InternalICs  ExternalResetVariant=Disabled  TRSumVariant=Passthrough  SumFdbkVariant=Disabled  SumVariant=Sum_PI  TsampFilterVariant=InternalTs  TsampNgainVariant=Passthrough  TsampIntegralVariant=Disabled_SignalSpec  ExternalSaturationOutDataTypeStr=Inherit: Same as second input  DerivativeSourceVariant=Disabled  PreIntVariant=InternalPreInt
  Product : Product
  Product1 : Product
  Saturation : Saturate  UpperLimit=200  LowerLimit=0
  Saturation1 : Saturate  UpperLimit=200  LowerLimit=0
  Step : Step  Time=0  After=0  SampleTime=0
  Step1 : Step  Time=600  Before=u0_2(1)  After=u0_2(1)+5  SampleTime=0
  Step2 : Step  Time=400  Before=u0_1(1)  After=u0_1(1)+5  SampleTime=0
  Step4 : Step  Time=6000  After=-0.1  SampleTime=0
  Step5 : Step  Time=7000  After=0.1  SampleTime=0
  Sum : Sum  Inputs=|+-
  Sum1 : Sum  Inputs=|+-
  Heat1 : Outport
  Heat2 : Outport  Port=2
  wires:
  Header Pressure/1 -> Sum/2
  Sum/1 -> PID Controller2/1  "error"
  Step2/1 -> Add/2  "Nominal Heat1"
  Step/1 -> Product/1, Product1/2
  MATLAB Function/1(Qsp1) -> Saturation1/1, Add2/1, Sum1/2  "Heat1"
  MATLAB Function/2(Qsp2) -> Saturation/1, Add2/2  "Heat2"
  Combustion Lag Boiler 1/1 -> Heat1/1
  Add/1 -> MATLAB Function/1(Q1_nom)
  Step1/1 -> Add1/2  "Nominal Heat2"
  Add1/1 -> MATLAB Function/2(Q2_nom)
  Add2/1 -> Gain1/1
  Gain1/1 -> Sum1/1
  Sum1/1 -> PID Controller/1
  Product1/1 -> Add/1, Gain/1
  PID Controller/1 -> Product1/1
  Combustion Lag Boiler 2/1 -> Heat2/1
  PID Controller2/1 -> Product/2
  Product/1 -> MATLAB Function/3(Q_bias)
  Constant/1 -> Add5/1  "Operating Header Pressure"
  Saturation/1 -> Combustion Lag Boiler 2/1  "Actuator Saturation2"
  Saturation1/1 -> Combustion Lag Boiler 1/1  "Actuator Saturation1"
  Add5/1 -> Sum/1
  Step5/1 -> Add5/2
  Step4/1 -> Add5/3
  Gain/1 -> Add1/1

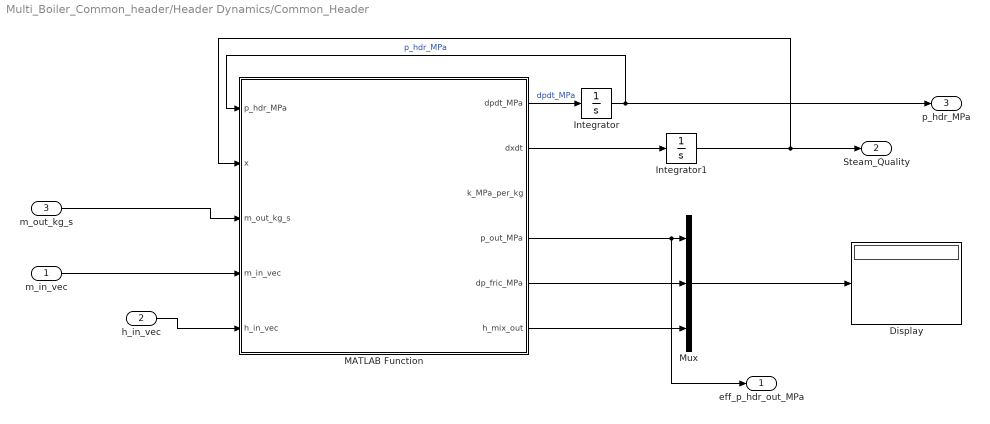
== system Multi_Boiler_Common_header/Header Dynamics/Common_Header ==
  m_in_vec : Inport
  h_in_vec : Inport  Port=2
  m_out_kg_s : Inport  Port=3
  Display : Display
  Integrator : Integrator  InitialCondition=8.5
  Integrator1 : Integrator  InitialCondition=0.082
  MATLAB Function : MATLAB Function  TreatAsAtomicUnit=on
  Mux : Mux  Inputs=3
  eff_p_hdr_out_MPa : Outport
  Steam_Quality : Outport  Port=2
  p_hdr_MPa : Outport  Port=3
  wires:
  m_in_vec/1 -> MATLAB Function/4(m_in_vec)
  h_in_vec/1 -> MATLAB Function/5(h_in_vec)
  m_out_kg_s/1 -> MATLAB Function/3(m_out_kg_s)
  MATLAB Function/1(dpdt_MPa) -> Integrator/1  "dpdt_MPa"
  MATLAB Function/2(dxdt) -> Integrator1/1
  Integrator/1 -> MATLAB Function/1(p_hdr_MPa), p_hdr_MPa/1  "p_hdr_MPa"
  Integrator1/1 -> MATLAB Function/2(x), Steam_Quality/1
  MATLAB Function/5(dp_fric_MPa) -> Mux/2
  MATLAB Function/4(p_out_MPa) -> eff_p_hdr_out_MPa/1, Mux/1
  MATLAB Function/6(h_mix_out) -> Mux/3
  Mux/1 -> Display/1

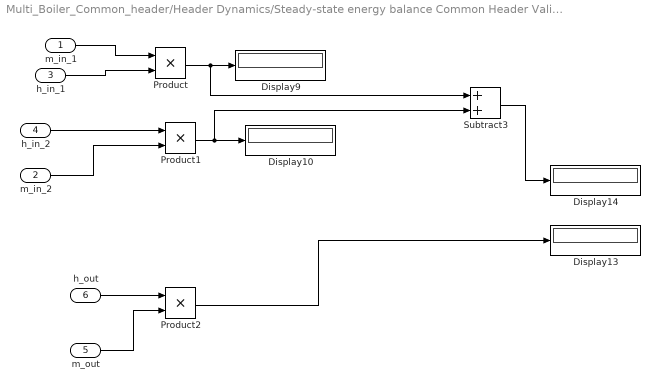
== system Multi_Boiler_Common_header/Header Dynamics/Steady‑state energy balance Common Header Validation ==
  m_in_1 : Inport
  m_in_2 : Inport  Port=2
  h_in_1 : Inport  Port=3
  h_in_2 : Inport  Port=4
  m_out : Inport  Port=5
  h_out : Inport  Port=6
  Display{9..10,13..14} (4 alike) : Display
  Product : Product
  Product1 : Product
  Product2 : Product
  Subtract3 : Sum
  wires:
  Subtract3/1 -> Display14/1
  Product1/1 -> Subtract3/2, Display10/1
  h_out/1 -> Product2/1
  Product/1 -> Subtract3/1, Display9/1
  m_in_2/1 -> Product1/2
  m_in_1/1 -> Product/1
  Product2/1 -> Display13/1
  h_in_1/1 -> Product/2
  h_in_2/1 -> Product1/1
  m_out/1 -> Product2/2

== system Multi_Boiler_Common_header/Header Dynamics/Steady‑state mass balance Common Header Validation ==
  m_in_1 : Inport
  m_in_2 : Inport  Port=2
  m_out : Inport  Port=3
  Add : Sum
  Display10 : Display
  Display9 : Display
  wires:
  m_in_1/1 -> Add/1
  Add/1 -> Display9/1
  m_out/1 -> Display10/1
  m_in_2/1 -> Add/2

== system Multi_Boiler_Common_header/Header Dynamics/Steam_Release_control_valve  ==
  p_up_MPa : Inport
  x_hdr : Inport  Port=2
  P_down_MPa : Inport  Port=3
  opening_out : Inport  Port=4
  MATLAB Function : MATLAB Function  TreatAsAtomicUnit=on
  mdot_out_kg_s : Outport
  h_out_kJkg : Outport  Port=2
  wires:
  p_up_MPa/1 -> MATLAB Function/1(p_up_MPa)
  x_hdr/1 -> MATLAB Function/2(x_hdr)
  P_down_MPa/1 -> MATLAB Function/3(P_down_MPa)
  opening_out/1 -> MATLAB Function/4(opening_out)
  MATLAB Function/1(mdot_out_kg_s) -> mdot_out_kg_s/1
  MATLAB Function/2(h_out_kJkg) -> h_out_kJkg/1

== system Multi_Boiler_Common_header/Valve1+pipe and Valve2/Boiler_Outlet_Valve2 ==
  p_up_MPa : Inport
  p_dn_MPa : Inport  Port=2
  opening : Inport  Port=3
  x_boiler : Inport  Port=4
  MATLAB Function : MATLAB Function  TreatAsAtomicUnit=on
  mdot_kg_s : Outport
  h_out_kJkg : Outport  Port=2
  regime : Outport  Port=3
  Tsat_C : Outport  Port=4
  dp_valve_MPa : Outport  Port=5
  x_out : Outport  Port=6
  wires:
  p_dn_MPa/1 -> MATLAB Function/2(p_dn_MPa)
  p_up_MPa/1 -> MATLAB Function/1(p_up_MPa)
  opening/1 -> MATLAB Function/3(opening)
  MATLAB Function/1(mdot_kg_s) -> mdot_kg_s/1
  MATLAB Function/2(h_out_kJkg) -> h_out_kJkg/1
  MATLAB Function/3(regime) -> regime/1
  MATLAB Function/4(Tsat_C) -> Tsat_C/1
  MATLAB Function/5(dp_valve_MPa) -> dp_valve_MPa/1
  x_boiler/1 -> MATLAB Function/4(x_boiler)
  MATLAB Function/6(x_out) -> x_out/1

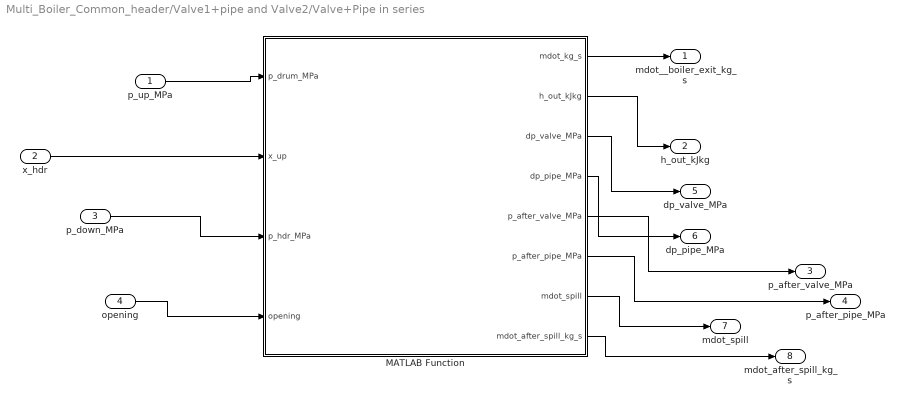
== system Multi_Boiler_Common_header/Valve1+pipe and Valve2/Valve+Pipe in series ==
  p_up_MPa : Inport
  x_hdr : Inport  Port=2
  p_down_MPa : Inport  Port=3
  opening : Inport  Port=4
  MATLAB Function : MATLAB Function  TreatAsAtomicUnit=on
  mdot__boiler_exit_kg_s : Outport
  h_out_kJkg : Outport  Port=2
  p_after_valve_MPa : Outport  Port=3
  p_after_pipe_MPa : Outport  Port=4
  dp_valve_MPa : Outport  Port=5
  dp_pipe_MPa : Outport  Port=6
  mdot_spill : Outport  Port=7
  mdot_after_spill_kg_s : Outport  Port=8
  wires:
  p_up_MPa/1 -> MATLAB Function/1(p_drum_MPa)
  x_hdr/1 -> MATLAB Function/2(x_up)
  p_down_MPa/1 -> MATLAB Function/3(p_hdr_MPa)
  opening/1 -> MATLAB Function/4(opening)
  MATLAB Function/1(mdot_kg_s) -> mdot__boiler_exit_kg_s/1
  MATLAB Function/2(h_out_kJkg) -> h_out_kJkg/1
  MATLAB Function/6(p_after_pipe_MPa) -> p_after_pipe_MPa/1
  MATLAB Function/5(p_after_valve_MPa) -> p_after_valve_MPa/1
  MATLAB Function/4(dp_pipe_MPa) -> dp_pipe_MPa/1
  MATLAB Function/3(dp_valve_MPa) -> dp_valve_MPa/1
  MATLAB Function/7(mdot_spill) -> mdot_spill/1
  MATLAB Function/8(mdot_after_spill_kg_s) -> mdot_after_spill_kg_s/1

== matlab function Multi_Boiler_Common_header/Valve1+pipe and Valve2/Valve+Pipe in series/MATLAB Function ==
  data: p_drum_MPa input; mdot_kg_s output; x_up input; p_hdr_MPa input; opening input; h_out_kJkg output; dp_valve_MPa output; dp_pipe_MPa output; p_after_valve_MPa output; p_after_pipe_MPa output; mdot_spill output; mdot_after_spill_kg_s output
function [mdot_kg_s, h_out_kJkg, dp_valve_MPa, dp_pipe_MPa, ...
          p_after_valve_MPa, p_after_pipe_MPa, mdot_spill, mdot_after_spill_kg_s] = ...
    SeriesValvePipe_HEM_DW_SC(p_drum_MPa, x_up, p_hdr_MPa, opening)


[mdot_kg_s, h_out_kJkg, dp_valve_MPa, dp_pipe_MPa, ...
          p_after_valve_MPa, p_after_pipe_MPa, mdot_spill, mdot_after_spill_kg_s] = ...
    SeriesValvePipe_HEM_DW_SC(p_drum_MPa, x_up, p_hdr_MPa, opening);

== matlab function Multi_Boiler_Common_header/Valve1+pipe and Valve2/Boiler_Outlet_Valve2/MATLAB Function ==
  data: p_up_MPa input; mdot_kg_s output; p_dn_MPa input; opening input; h_out_kJkg output; regime output; Tsat_C output; dp_valve_MPa output; x_boiler input; x_out output
function [mdot_kg_s, h_out_kJkg, regime, Tsat_C, dp_valve_MPa, x_out] = ...
    valve_boiler_to_header(p_up_MPa, p_dn_MPa, opening, x_boiler)


 [mdot_kg_s, h_out_kJkg, regime, Tsat_C, dp_valve_MPa, x_out] = ...
    valve_boiler_to_header(p_up_MPa, p_dn_MPa, opening, x_boiler);

== matlab function Multi_Boiler_Common_header/Header Dynamics/Common_Header/MATLAB Function ==
  data: p_hdr_MPa input; dpdt_MPa output size=[1 1]; x input; m_out_kg_s input; m_in_vec input; h_in_vec input; dxdt output size=[1 1]; k_MPa_per_kg output; p_out_MPa output; dp_fric_MPa output; h_mix_out output
function [dpdt_MPa, dxdt, k_MPa_per_kg, p_out_MPa, dp_fric_MPa, h_mix_out] = ...
    Header_NIn1Out_MPa_SC_TYPED(p_hdr_MPa, x, m_out_kg_s, m_in_vec, h_in_vec)



[dpdt_MPa, dxdt, k_MPa_per_kg, p_out_MPa, dp_fric_MPa, h_mix_out] = ...
    Header_NIn1Out_MPa_SC_TYPED(p_hdr_MPa, x, m_out_kg_s, m_in_vec, h_in_vec);

== matlab function Multi_Boiler_Common_header/Header Dynamics/Steam_Release_control_valve /MATLAB Function ==
  data: p_up_MPa input; mdot_out_kg_s output; x_hdr input; P_down_MPa input; opening_out input; h_out_kJkg output
function [mdot_out_kg_s, h_out_kJkg] = Valve_HeaderToLoad_HEM( ...
    p_up_MPa, x_hdr, P_down_MPa, opening_out)


[mdot_out_kg_s, h_out_kJkg] = Valve_HeaderToLoad_HEM( ...
    p_up_MPa, x_hdr, P_down_MPa, opening_out);

== matlab function Multi_Boiler_Common_header/Controller/Level Control Subsystem/MATLAB Function ==
  data: m input; q_f output
function q_f = feedwater_valve_boiler1(m)


q_f = feedwater_valve_boiler1(m);

== matlab function Multi_Boiler_Common_header/Controller/Level Control Subsystem/MATLAB Function1 ==
  data: m input; q_f output
function q_f = feedwater_valve_boiler2(m)


q_f = feedwater_valve_boiler2(m);

== matlab function Multi_Boiler_Common_header/Controller/Pressure Control/MATLAB Function ==
  data: Q1_nom input; Qsp1 output; Q2_nom input; Q_bias input; Qsp2 output
function [Qsp1, Qsp2] = allocator(Q1_nom, Q2_nom, Q_bias)

w1 = 0.5;
w2 = 0.5;
    Qsp1 = Q1_nom + w1*Q_bias;
    Qsp2 = Q2_nom + w2*Q_bias;
end

== matlab function Multi_Boiler_Common_header/Boilers/Boiler1/MATLAB Function ==
  data: Vwt input; DrumWaterLevel output; p_MPa input; ar input; Vsd input; WaterLevelDeviation output; av_out output; WaterLevelContribution output; SteamLevelContribution output
function [DrumWaterLevel, WaterLevelDeviation, av_out, WaterLevelContribution, SteamLevelContribution] = drum_level(Vwt, p_MPa, ar, Vsd)


[DrumWaterLevel, WaterLevelDeviation, av_out, WaterLevelContribution, SteamLevelContribution] = calculate_level(Vwt, p_MPa, ar, Vsd)

== matlab function Multi_Boiler_Common_header/Boilers/Boiler1/boiler_dynamics ==
  data: x input size=[4 1]; u input size=[4 1]; b input size=[1 1]; k input size=[1 1]; Vr input size=[1 1]; Adc input size=[1 1]; m_metal input size=[1 1]; m_riser input size=[1 1]; dxdt output size=[4 1]; tau_s input size=[1 1]; additional_outputs output size=[6 1]
function [dxdt, additional_outputs] = boiler(x, u, b, k, Vr, Adc, m_metal, m_riser, tau_s)
%#codegen
% Wrapper that calls the external boiler dynamics function.
[dxdt, additional_outputs] = boiler_dynamics_block( ...
    x, u, b, k, Vr, Adc, m_metal, m_riser, tau_s );

== matlab function Multi_Boiler_Common_header/Boilers/Boiler2/MATLAB Function ==
  data: Vwt input; DrumWaterLevel output; p_MPa input; ar input; Vsd input; WaterLevelDeviation output; av_out output; WaterLevelContribution output; SteamLevelContribution output
function [DrumWaterLevel, WaterLevelDeviation, av_out, WaterLevelContribution, SteamLevelContribution] = drum_level(Vwt, p_MPa, ar, Vsd)


[DrumWaterLevel, WaterLevelDeviation, av_out, WaterLevelContribution, SteamLevelContribution] = calculate_level(Vwt, p_MPa, ar, Vsd);

== matlab function Multi_Boiler_Common_header/Boilers/Boiler2/boiler_dynamics ==
  data: x input size=[4 1]; u input size=[4 1]; b input size=[1 1]; k input size=[1 1]; Vr input size=[1 1]; Adc input size=[1 1]; m_metal input size=[1 1]; m_riser input size=[1 1]; dxdt output size=[4 1]; tau_s input size=[1 1]; additional_outputs output size=[6 1]
function [dxdt, additional_outputs] = boiler(x, u, b, k, Vr, Adc, m_metal, m_riser, tau_s)
%#codegen
% Wrapper that calls the external boiler dynamics function.
[dxdt, additional_outputs] = boiler_dynamics_block( ...
    x, u, b, k, Vr, Adc, m_metal, m_riser, tau_s );
